simulink model "untitled"  (R2020b)
settings: Solver=VariableStepAuto  StartTime=0.0  StopTime=1  RelTol=1e-3
values from neighbouring files (symbols this model uses):
  C1 = (Kp + (tf([1 1], [1 -1], T)*Ki*T/2))    [projCD.m]
  C2 = (tf([1 -1], [1 0], T)*Kd/T)    [projCD.m]
  F = tf([a0], [1 w0/Q w0^2])    [projCD.m]
  G = tf([75], conv([1 10], [1 15]))    [projCD.m]
  Gpid = (Kp + (tf([1 1], [1 -1], T)*Ki*T/2) + (tf([1 -1], [1 0], T)*Kd/T))    [projCD.m]
  T = 11e-3    (= 0.011)    [projCD.m]
settings Model: Creator=Erick  LastModifiedBy=Erick

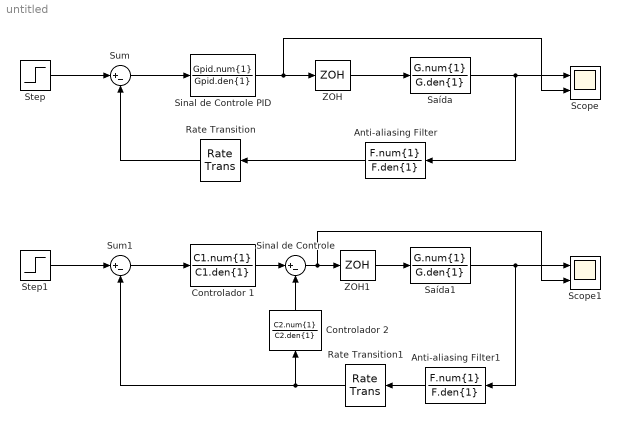
== system untitled ==
  Anti-aliasing Filter : TransferFcn  Numerator=F.num{1}  Denominator=F.den{1}
  Anti-aliasing Filter1 : TransferFcn  Numerator=F.num{1}  Denominator=F.den{1}
  Controlador 1 : DiscreteTransferFcn  Numerator=C1.num{1}  Denominator=C1.den{1}  SampleTime=T
  Controlador 2 : DiscreteTransferFcn  Numerator=C2.num{1}  Denominator=C2.den{1}  SampleTime=T
  Rate Transition : RateTransition  OutPortSampleTime=T
  Rate Transition1 : RateTransition  OutPortSampleTime=T
  Saída : TransferFcn  Numerator=G.num{1}  Denominator=G.den{1}
  Saída1 : TransferFcn  Numerator=G.num{1}  Denominator=G.den{1}
  Scope : Scope  NumInputPorts=2
  Scope1 : Scope  NumInputPorts=2
  Sinal de Controle : Sum  Inputs=|+-
  Sinal de Controle PID : DiscreteTransferFcn  Numerator=Gpid.num{1}  Denominator=Gpid.den{1}  SampleTime=T
  Step : Step  Time=0  SampleTime=0
  Step1 : Step  Time=0  SampleTime=0
  Sum : Sum  Inputs=|+-
  Sum1 : Sum  Inputs=|+-
  ZOH : ZeroOrderHold  SampleTime=T
  ZOH1 : ZeroOrderHold  SampleTime=T
  wires:
  ZOH/1 -> Saída/1
  Sinal de Controle PID/1 -> Scope/2, ZOH/1
  Saída/1 -> Anti-aliasing Filter/1, Scope/1
  Sum/1 -> Sinal de Controle PID/1
  Step/1 -> Sum/1
  Anti-aliasing Filter/1 -> Rate Transition/1
  Rate Transition/1 -> Sum/2
  Saída1/1 -> Anti-aliasing Filter1/1, Scope1/1
  Sum1/1 -> Controlador 1/1
  ZOH1/1 -> Saída1/1
  Step1/1 -> Sum1/1
  Rate Transition1/1 -> Controlador 2/1, Sum1/2
  Controlador 1/1 -> Sinal de Controle/1
  Sinal de Controle/1 -> Scope1/2, ZOH1/1
  Controlador 2/1 -> Sinal de Controle/2
  Anti-aliasing Filter1/1 -> Rate Transition1/1
